simulink model "Vehicle_Parked_Condition"  (R2019a)
settings: Solver=FixedStepDiscrete  StartTime=0.0  StopTime=10.0  FixedStep=0.08  RelTol=1e-3
values from neighbouring files (symbols this model uses):
  Ignition = timeseries    [TT1_in.m]
undefined symbols (not defined in the file or in its folder): Day_Night_Chk, Delay, Light, Lock, Sample_Time, Terminate
libraries: simulink x10
settings Model: Creator=Shivansh  LastModifiedBy=vmadmin
settings DataIOCC: ReturnWorkspaceOutputs=off
settings OptimizationCC: DefaultParameterBehavior=Inlined  UseDivisionForNetSlopeComputation=UseDivisionForReciprocalsOfIntegersOnly  EnhancedBackFolding=on  PassReuseOutputArgsAs=Individual arguments  OptimizeBlockOrder=speed  DifferentSizesBufferReuse=on  OptimizationCustomize=off
settings DebuggingCC: SignalInfNanChecking=warning  ParameterTunabilityLossMsg=error  UniqueDataStoreMsg=warning  AssertControl=DisableAll  PregeneratedLibrarySubsystemCodeDiagnostic=none  StrictBusMsg=ErrorOnBusTreatedAsVector  ArithmeticOperatorsInVariantConditions=warning
settings SFSimCC: SimUseLocalCustomCode=off  MATLABDynamicMemAlloc=off
settings RTWCC: SystemTargetFile=ert.tlc  TemplateMakefile=ert_default_tmf  GenerateReport=on  RTWUseLocalCustomCode=off  IncludeHyperlinkInReport=on  LaunchReport=on  GenerateTraceInfo=on  GenerateTraceReport=on  GenerateTraceReportSl=on  GenerateTraceReportSf=on  GenerateTraceReportEml=on
settings CodeAppCC: ForceParamTrailComments=on  IgnoreCustomStorageClasses=off  OperatorAnnotations=on  SimulinkDataObjDesc=on  SFDataObjDesc=on  InsertBlockDesc=on
settings ERTTargetCC: TargetLangStandard=C99 (ISO)  CodeReplacementLibrary=AUTOSAR 4.0  UtilityFuncGeneration=Shared location  GenerateSampleERTMain=on  SupportNonFinite=off  ParenthesesLevel=Maximum  CastingMode=Standards  GenerateSharedConstants=off  InlinedParameterPlacement=NonHierarchical  ERTCustomFileTemplate=example_file_process.tlc  EnableSignedLeftShifts=off  EnableSignedRightShifts=off

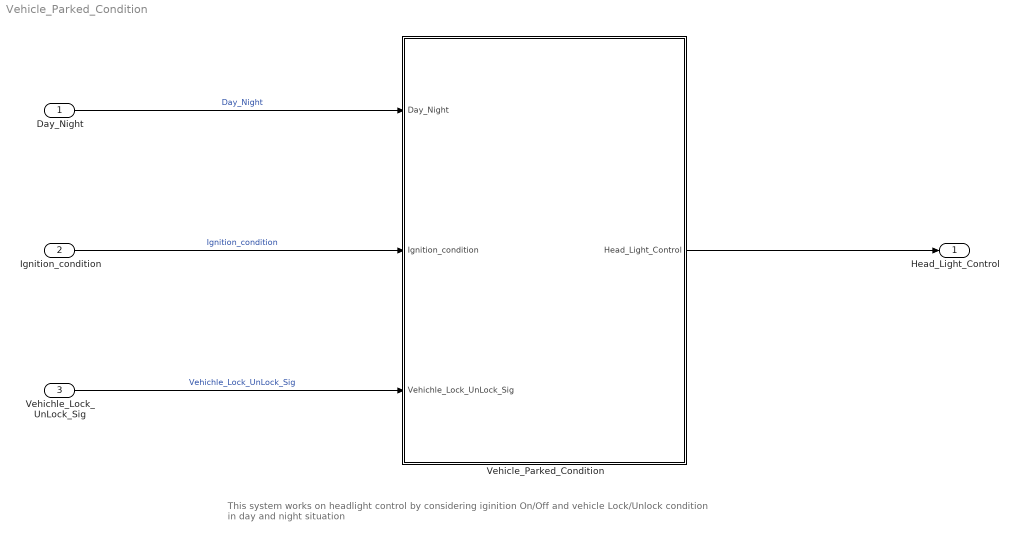
== system Vehicle_Parked_Condition ==
  note: This system works on headlight control by considering iginition On/Off and vehicle Lock/Unlock condition in day and night situation
  Day_Night : Inport
  Ignition_condition : Inport  Port=2
  Vehichle_Lock_UnLock_Sig : Inport  Port=3
  Vehicle_Parked_Condition : Subsystem
  Head_Light_Control : Outport  VectorParamsAs1DForOutWhenUnconnected=on
  wires:
  Vehicle_Parked_Condition/1(Head_Light_Control) -> Head_Light_Control/1
  Day_Night/1 -> Vehicle_Parked_Condition/1(Day_Night)  "Day_Night"
  Vehichle_Lock_UnLock_Sig/1 -> Vehicle_Parked_Condition/3(Vehichle_Lock_UnLock_Sig)  "Vehichle_Lock_UnLock_Sig"
  Ignition_condition/1 -> Vehicle_Parked_Condition/2(Ignition_condition)  "Ignition_condition"

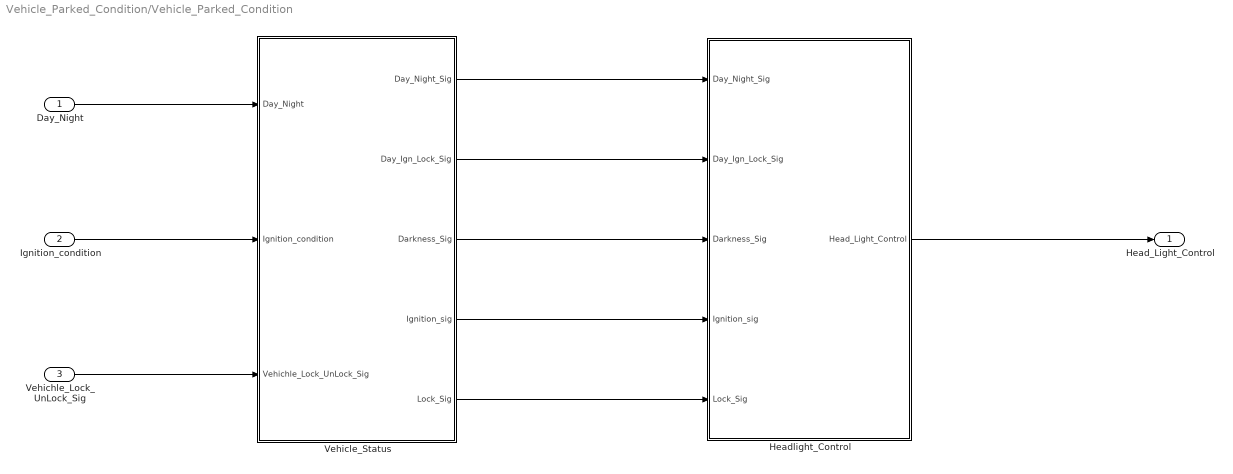
== system Vehicle_Parked_Condition/Vehicle_Parked_Condition ==
  Day_Night : Inport
  Ignition_condition : Inport  Port=2
  Vehichle_Lock_UnLock_Sig : Inport  Port=3
  Headlight_Control : Subsystem
  Vehicle_Status : Subsystem
  Head_Light_Control : Outport  VectorParamsAs1DForOutWhenUnconnected=on
  wires:
  Vehicle_Status/5(Lock_Sig) -> Headlight_Control/5(Lock_Sig)
  Vehicle_Status/4(Ignition_sig) -> Headlight_Control/4(Ignition_sig)
  Vehicle_Status/1(Day_Night_Sig) -> Headlight_Control/1(Day_Night_Sig)
  Vehicle_Status/2(Day_Ign_Lock_Sig) -> Headlight_Control/2(Day_Ign_Lock_Sig)
  Vehicle_Status/3(Darkness_Sig) -> Headlight_Control/3(Darkness_Sig)
  Day_Night/1 -> Vehicle_Status/1(Day_Night)
  Headlight_Control/1(Head_Light_Control) -> Head_Light_Control/1
  Ignition_condition/1 -> Vehicle_Status/2(Ignition_condition)
  Vehichle_Lock_UnLock_Sig/1 -> Vehicle_Status/3(Vehichle_Lock_UnLock_Sig)

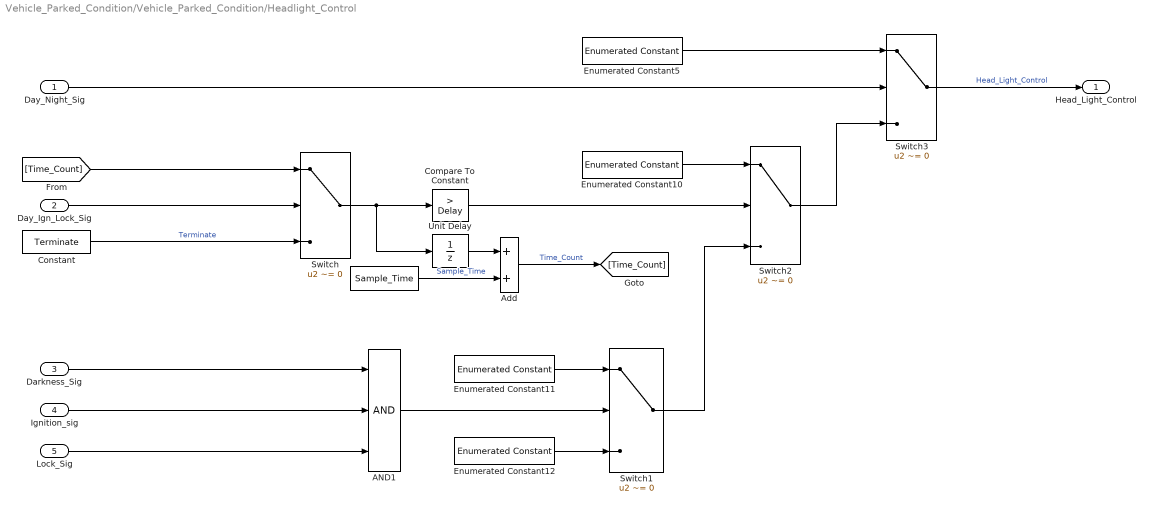
== system Vehicle_Parked_Condition/Vehicle_Parked_Condition/Headlight_Control ==
  Day_Night_Sig : Inport
  Day_Ign_Lock_Sig : Inport  Port=2
  Darkness_Sig : Inport  Port=3
  Ignition_sig : Inport  Port=4
  Lock_Sig : Inport  Port=5
  " " : Constant  Value=Sample_Time
  AND1 : Logic  Inputs=3  AllPortsSameDT=off  OutDataTypeStr=boolean
  Add : Sum
  Compare To Constant : simulink/Logic and Bit Operations/Compare To Constant  relop=>  const=Delay  OutDataTypeStr=boolean
  Constant : Constant  Value=Terminate
  Enumerated Constant10 : simulink/Sources/Enumerated Constant  OutDataTypeStr=Enum: Light  Value=Light.Headlight_Off  SampleTime=inf
      settings: SourceProductName=Simulink
  Enumerated Constant11 : simulink/Sources/Enumerated Constant  OutDataTypeStr=Enum: Light  Value=Light.Low_Beam  SampleTime=inf
      settings: SourceProductName=Simulink
  Enumerated Constant12 : simulink/Sources/Enumerated Constant  OutDataTypeStr=Enum: Light  Value=Light.Low_Beam  SampleTime=inf
      settings: SourceProductName=Simulink
  Enumerated Constant5 : simulink/Sources/Enumerated Constant  OutDataTypeStr=Enum: Light  Value=Light.Headlight_Off  SampleTime=inf
      settings: SourceProductName=Simulink
  Switch : Switch  Criteria=u2 ~= 0
  Switch1 : Switch  Criteria=u2 ~= 0
  Switch2 : Switch  Criteria=u2 ~= 0
  Switch3 : Switch  Criteria=u2 ~= 0  OutDataTypeStr=Inherit: Inherit via back propagation
  Unit Delay : UnitDelay  SampleTime=-1  HasFrameUpgradeWarning=on
  Head_Light_Control : Outport  VectorParamsAs1DForOutWhenUnconnected=on
  wires:
  Enumerated Constant11/1 -> Switch1/1
  Day_Ign_Lock_Sig/1 -> Switch/2
  Day_Night_Sig/1 -> Switch3/2
  Switch1/1 -> Switch2/3
  Darkness_Sig/1 -> AND1/1
  Switch2/1 -> Switch3/3
  Enumerated Constant12/1 -> Switch1/3
  Unit Delay/1 -> Add/1
  Enumerated Constant10/1 -> Switch2/1
  Enumerated Constant5/1 -> Switch3/1
  " "/1 -> Add/2  "Sample_Time"
  Lock_Sig/1 -> AND1/3
  Switch/1 -> Unit Delay/1, Compare To Constant/1
  AND1/1 -> Switch1/2
  Compare To Constant/1 -> Switch2/2
  Switch3/1 -> Head_Light_Control/1  "Head_Light_Control"
  Ignition_sig/1 -> AND1/2
  Add/1 -> [Time_Count]  "Time_Count"
  [Time_Count] -> Switch/1
  Constant/1 -> Switch/3  "Terminate"

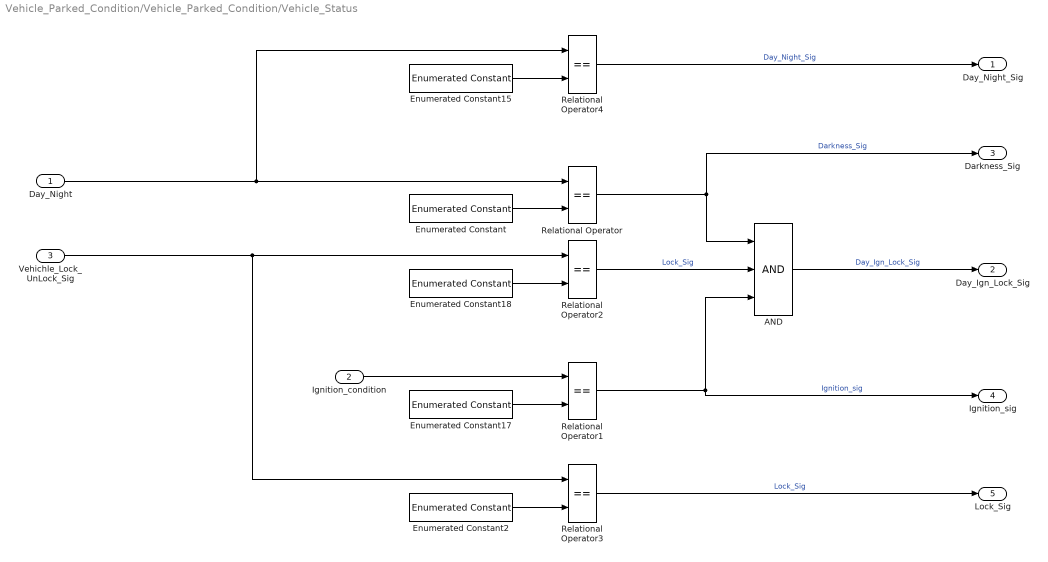
== system Vehicle_Parked_Condition/Vehicle_Parked_Condition/Vehicle_Status ==
  Day_Night : Inport
  Ignition_condition : Inport  Port=2
  Vehichle_Lock_UnLock_Sig : Inport  Port=3
  AND : Logic  Inputs=3  AllPortsSameDT=off  OutDataTypeStr=boolean
  Enumerated Constant : simulink/Sources/Enumerated Constant  OutDataTypeStr=Enum: Day_Night_Chk  Value=Day_Night_Chk.Darkness  SampleTime=inf
      settings: SourceProductName=Simulink
  Enumerated Constant15 : simulink/Sources/Enumerated Constant  OutDataTypeStr=Enum: Day_Night_Chk  Value=Day_Night_Chk.Day_Time  SampleTime=inf
      settings: SourceProductName=Simulink
  Enumerated Constant17 : simulink/Sources/Enumerated Constant  OutDataTypeStr=Enum: Ignition  Value=Ignition.Ignition_Off  SampleTime=inf
      settings: SourceProductName=Simulink
  Enumerated Constant18 : simulink/Sources/Enumerated Constant  OutDataTypeStr=Enum: Lock  Value=Lock.Vehicle_locked  SampleTime=inf
      settings: SourceProductName=Simulink
  Enumerated Constant2 : simulink/Sources/Enumerated Constant  OutDataTypeStr=Enum: Lock  Value=Lock.Vehicle_locked  SampleTime=inf
      settings: SourceProductName=Simulink
  Relational Operator{,1..4} (5 alike) : RelationalOperator  Operator===  OutDataTypeStr=boolean  RndMeth=Simplest
  Day_Night_Sig : Outport  VectorParamsAs1DForOutWhenUnconnected=on
  Day_Ign_Lock_Sig : Outport  Port=2  VectorParamsAs1DForOutWhenUnconnected=on
  Darkness_Sig : Outport  Port=3  VectorParamsAs1DForOutWhenUnconnected=on
  Ignition_sig : Outport  Port=4  VectorParamsAs1DForOutWhenUnconnected=on
  Lock_Sig : Outport  Port=5  VectorParamsAs1DForOutWhenUnconnected=on
  wires:
  Enumerated Constant18/1 -> Relational Operator2/2
  Enumerated Constant/1 -> Relational Operator/2
  Enumerated Constant2/1 -> Relational Operator3/2
  Enumerated Constant15/1 -> Relational Operator4/2
  Relational Operator1/1 -> AND/3, Ignition_sig/1  "Ignition_sig"
  Relational Operator/1 -> AND/1, Darkness_Sig/1  "Darkness_Sig"
  Vehichle_Lock_UnLock_Sig/1 -> Relational Operator2/1, Relational Operator3/1
  Day_Night/1 -> Relational Operator/1, Relational Operator4/1
  Enumerated Constant17/1 -> Relational Operator1/2
  AND/1 -> Day_Ign_Lock_Sig/1  "Day_Ign_Lock_Sig"
  Ignition_condition/1 -> Relational Operator1/1
  Relational Operator3/1 -> Lock_Sig/1  "Lock_Sig"
  Relational Operator4/1 -> Day_Night_Sig/1  "Day_Night_Sig"
  Relational Operator2/1 -> AND/2  "Lock_Sig"
